simulink model "Model_01_Position_Signal"  (R2020a)
settings: Solver=ode4  StartTime=0.0  StopTime=2  FixedStep=1e-4  RelTol=1e-3
settings Model: Creator=samee  LastModifiedBy=DEVIKAT
settings DebuggingCC: UnconnectedInputMsg=none  UnconnectedOutputMsg=none  UnconnectedLineMsg=none

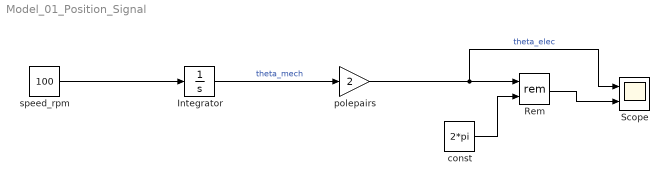
== system Model_01_Position_Signal ==
  Integrator : Integrator
  Rem : Math  Operator=rem  SaturateOnIntegerOverflow=on
  Scope : Scope  NumInputPorts=2
  const : Constant  Value=2*pi
  polepairs : Gain  Gain=2
  speed_rpm : Constant  Value=100
  wires:
  Integrator/1 -> polepairs/1  "theta_mech"
  polepairs/1 -> Scope/1, Rem/1  "theta_elec"
  const/1 -> Rem/2
  Rem/1 -> Scope/2
  speed_rpm/1 -> Integrator/1
